simulink model "pitch_thrust_input_model"  (R2015a)
settings: Solver=ode45  SolverMode=SingleTasking  StartTime=0.0  StopTime=120  FixedStep=0.01  RelTol=1e-6
undefined symbols (not defined in the file or in its folder): T
settings Model: Creator=Andrew  LastModifiedBy=Andrew
settings OptimizationCC: BlockReduction=off  BooleanDataType=off
settings DebuggingCC: SaveWithParameterizedLinksMsg=none  UnderspecifiedInitializationDetection=Classic  MergeDetectMultiDrivingBlocksExec=none  SignalResolutionControl=TryResolveAllWithWarning
settings HardwareCC: TargetUnknown=on

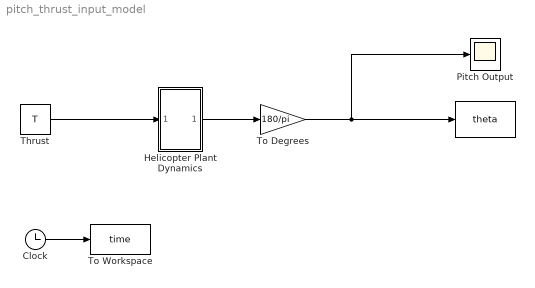
== system pitch_thrust_input_model ==
  "   " : ToWorkspace  VariableName=theta  SampleTime=-1
      settings: Save2DSignal=2-D array (concatenate along first dimension)
  Clock : Clock
  Helicopter Plant Dynamics : Subsystem
  Pitch Output : Scope
      settings: TimeRange=120  YMin=-100  YMax=700  SaveName=theta_step_cl
  Thrust : Constant  Value=T
  "To Degrees " : Gain  Gain=180/pi
  To Workspace : ToWorkspace  VariableName=time  SampleTime=-1
      settings: Save2DSignal=2-D array (concatenate along first dimension)
  wires:
  Clock/1 -> To Workspace/1
  Helicopter Plant Dynamics/1(Out1) -> "To Degrees "/1
  Thrust/1 -> Helicopter Plant Dynamics/1(In1)
  "To Degrees "/1 -> "   "/1, Pitch Output/1

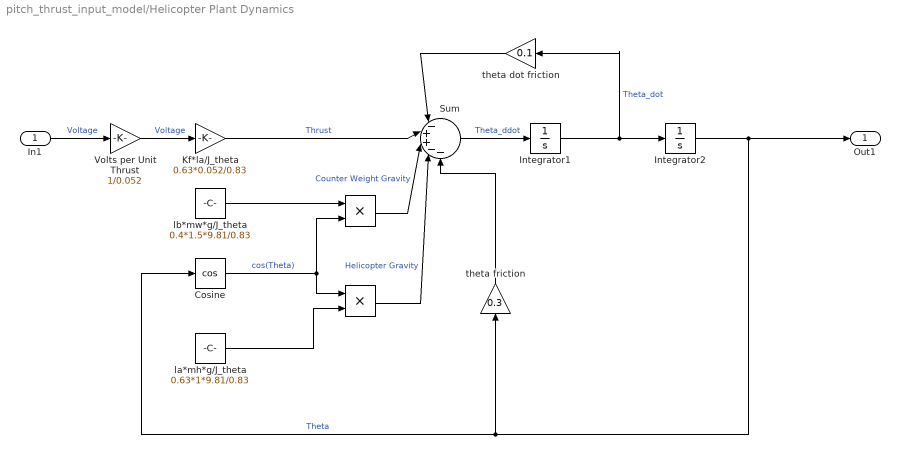
== system pitch_thrust_input_model/Helicopter Plant Dynamics ==
  In1 : Inport
  " " : Product
  "  " : Product
  Cosine : Trigonometry  Operator=cos
  Integrator1 : Integrator
  Integrator2 : Integrator  InitialCondition=-pi/8
  Kf*la/J_theta : Gain  Gain=0.63*0.052/0.83
  Sum : Sum  Inputs=|-++--
  Volts per Unit Thrust : Gain  Gain=1/0.052
  la*mh*g/J_theta : Constant  Value=0.63*1*9.81/0.83
  lb*mw*g/J_theta : Constant  Value=0.4*1.5*9.81/0.83
  theta friction : Gain  Gain=0.3
  theta dot friction : Gain  Gain=0.1
  Out1 : Outport
  wires:
  Volts per Unit Thrust/1 -> Kf*la/J_theta/1  "Voltage"
  Integrator1/1 -> Integrator2/1, theta dot friction/1  "Theta_dot"
  Integrator2/1 -> Cosine/1, theta friction/1, Out1/1  "Theta"
  Kf*la/J_theta/1 -> Sum/2  "Thrust"
  Cosine/1 -> " "/2, "  "/1  "cos(Theta)"
  la*mh*g/J_theta/1 -> "  "/2
  lb*mw*g/J_theta/1 -> " "/1
  "  "/1 -> Sum/4  "Helicopter Gravity"
  Sum/1 -> Integrator1/1  "Theta_ddot"
  " "/1 -> Sum/3  "Counter Weight Gravity"
  theta dot friction/1 -> Sum/1
  theta friction/1 -> Sum/5
  In1/1 -> Volts per Unit Thrust/1  "Voltage"
